simulink model "solar"  (Simulink 7.7)
settings: Solver=ode23t  StartTime=0.0  StopTime=10  RelTol=1e-3
PreLoadFcn:
  | load elec_solar_iv_data.mat;
  | idx_data = 2;
undefined symbols (not defined in the file): iv_data
libraries: fl_lib x4, nesl_utility x3, elec_lib x2
Description:
  | Solar Cell Parameter Tuning
  | 
  | This demo optimizes the Solar Cell block's parameters to fit data defined over
  | a range of different temperatures. It uses the MATLAB(R) optimization function
  | fminsearch. Other products available for performing this type of parameter
  | fitting with SimElectronics(TM) models are the Optimization Toolbox(TM) and
  | the Simulink(R) Design Optimization(TM). These products provide predefined
  | functions to manipulate and analyze blocks using GUIs or a command line approach.
  | 
  | Copyright 2008-2011 The MathWorks, Inc.
settings Model: Creator=MathWorks  LastModifiedBy=Vikas
settings DataIOCC: LimitDataPoints=off  SaveTime=off  OutputOption=SpecifiedOutputTimes  OutputTimes=[iv_data(idx_data).v/iv_data(idx_data).v(end)]
settings DebuggingCC: SolverPrmCheckMsg=none  StrictBusMsg=Warning

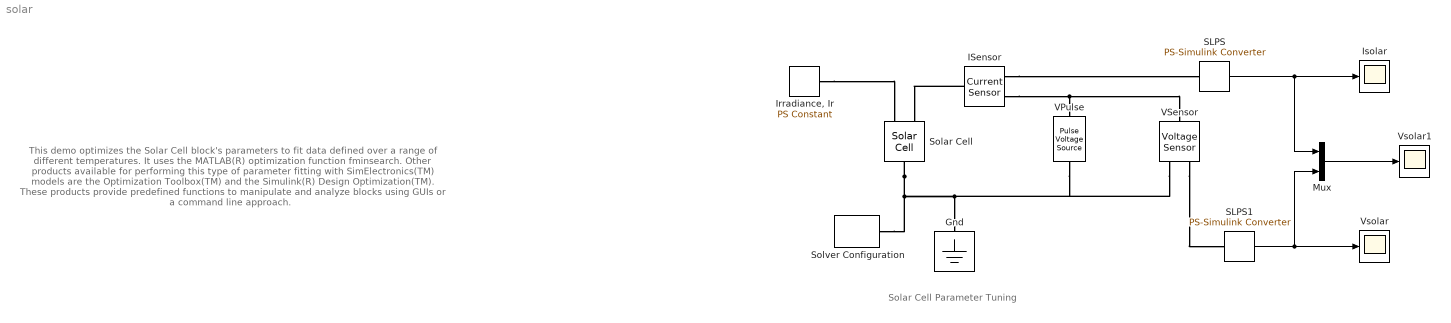
== system solar ==
  note: Solar Cell Parameter Tuning
  note: This demo optimizes the Solar Cell block's parameters to fit data defined over
      | a range of different temperatures. It uses the MATLAB(R) optimization function
      | fminsearch. Other products available for performing this type of parameter
      | fitting with SimElectronics(TM) models are the Optimization Toolbox(TM) and
      | the Simulink(R) Design Optimization(TM). These products provide predefined
      | functions to manipulate and analyze blocks using GUIs or a command line approach.
  Gnd : fl_lib/Electrical/Electrical Elements/Electrical Reference  SystemSampleTime=-1  i_Log=off  LocalVarNames=|i  LocalVarDescs=|i  LocalVarLogging=[]
  ISensor : fl_lib/Electrical/Electrical Sensors/Current Sensor  SystemSampleTime=-1  i1_Log=off  v1_Log=off  LocalVarNames=|i1|v1  LocalVarDescs=|i1|v1  LocalVarLogging=[0 0]
  "Irradiance, Ir" : fl_lib/Physical Signals/Sources/PS Constant  SystemSampleTime=-1  constant=1000  LocalVarLogging=[]
  Isolar : Scope
      settings: TimeRange=1  YMin=2  YMax=8  SaveName=Io
  Mux : Mux  Inputs=2
  SLPS : nesl_utility/PS-Simulink Converter  SystemSampleTime=-1  PhysicalDomain=network_engine_domain  LeftPortType=input  RightPortType=output  SubClassName=ps_output  Unit=1  AffineConversion=off
  SLPS1 : nesl_utility/PS-Simulink Converter  SystemSampleTime=-1  PhysicalDomain=network_engine_domain  LeftPortType=input  RightPortType=output  SubClassName=ps_output  Unit=1  AffineConversion=off
  Solar Cell : elec_lib/Sources/Solar Cell  SystemSampleTime=-1  prm=1  Isc=7.34 A  Voc=0.6 V  Is=1e-06 A  Is2=0 A  Iph=7.34 A  Ir0=1000 W/m^2  ec=1.5  N2=2  Rs=0 Ohm  Rp=Inf Ohm  TIPH1=0 1/K  EG=1.11 eV  TXIS1=3  TXIS2=3  TRS1=0  TRP1=0  TFIXED=iv_data(idx_data).temperature C  Tmeas=25 C  LocalVarLogging=[]
  Solver Configuration : nesl_utility/Solver Configuration  SystemSampleTime=-1  PhysicalDomain=network_engine_domain  LeftPortType=input  RightPortType=generic  SubClassName=solver  Accelerate=off  Profile=off  ResidualTolerance=1e-9  MaxNonlinIter=3  MaxModeIter=2  DoFixedCost=off  UseLocalSampling=off  DoDC=off  LinearAlgebra=Sparse  LocalSolverSampleTime=.001  LocalSolverChoice=NE_BACKWARD_EULER_ADVANCER  UseLocalSolver=off
  VPulse : elec_lib/Additional Components/SPICE-Compatible Components/Sources/Pulse Voltage Source  SystemSampleTime=-1  V1=0 V  V2=iv_data(idx_data).v(end) V  TD=0 s  TR=1 s  TF=0 s  PW=Inf s  PER=Inf s  voltage_Log=off  LocalVarNames=|voltage  LocalVarDescs=|Voltage (V)  LocalVarLogging=0
  VSensor : fl_lib/Electrical/Electrical Sensors/Voltage Sensor  SystemSampleTime=-1  i1_Log=off  v1_Log=off  LocalVarNames=|i1|v1  LocalVarDescs=|i1|v1  LocalVarLogging=[0 0]
  Vsolar : Scope
      settings: TimeRange=1  YMin=0  YMax=0.8  SaveName=Vo
  Vsolar1 : Scope
      settings: TimeRange=1  YMin=0  YMax=0.8  SaveName=Vo1
  wires:
  SLPS/1 -> Isolar/1, Mux/1
  SLPS1/1 -> Vsolar/1, Mux/2
  Mux/1 -> Vsolar1/1
  connections:
  "Irradiance, Ir"/RConn1 -- Solar Cell/LConn1
  ISensor/LConn1 -- Solar Cell/LConn2
  Solar Cell/RConn1 -- Gnd/LConn1 -- VPulse/RConn1 -- VSensor/RConn2 -- Solver Configuration/RConn1
  ISensor/RConn1 -- SLPS/LConn1
  ISensor/RConn2 -- VPulse/LConn1 -- VSensor/LConn1
  VSensor/RConn1 -- SLPS1/LConn1
